simulink model "IM_model"  (R2021a)
settings: Solver=FixedStepAuto  StartTime=0.0  StopTime=40  FixedStep=1e-5  RelTol=1e-3
InitFcn:
  | parameter
values from neighbouring files (symbols this model uses):
  f = 60    [parameter.m]
  Jm = 242.28    [parameter.m]
  L1 = X1/2/pi/f    (= 3.36819606065e-05)    [parameter.m]
  L1a = X1a/2/pi/f    (= 6.73639212131e-05)    [parameter.m]
  L2 = X2/2/pi/f    (= 2.99288217902e-05)    [parameter.m]
  L2a = X2a/2/pi/f    (= 6.41561024441e-05)    [parameter.m]
  Power = 4300e3    (= 4300000)    [parameter.m]
  pp = pole/2    (= 3)    [parameter.m]
  R1 = 0.000789831    [parameter.m]
  R1a = 2*R1    (= 0.001579662)    [parameter.m]
  R2 = 0.00052717    [parameter.m]
  R2a = 2*R2/0.933    (= 0.00113005359057)    [parameter.m]
  Vll = 700    [parameter.m]
libraries: spsACVoltageSourceLib x9, spsFourierLib x3, spsAsynchronousMachineSIUnitsLib x3, spsVoltageMeasurementLib x3, eeStairGenerator x1, spspowerguiLib x1
settings Model: Creator=enes_  LastModifiedBy=enes_

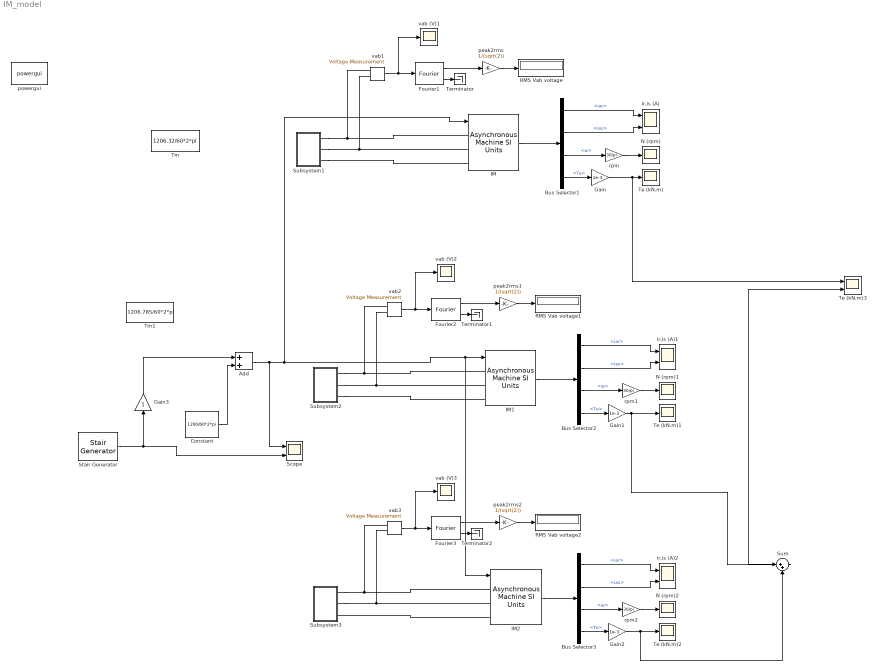
== system IM_model ==
  Add : Sum
  Bus Selector1 : BusSelector  OutputSignals=iar,ias,w,Te
  Bus Selector2 : BusSelector  OutputSignals=iar,ias,w,Te
  Bus Selector3 : BusSelector  OutputSignals=iar,ias,w,Te
  Constant : Constant  Value=1200/60*2*pi
  Fourier1 : spsFourierLib/Fourier  Freq=60  n=1  InInit=[0, 0]  Ts=0
      settings: SourceProductBaseCode=PS
  Fourier2 : spsFourierLib/Fourier  Freq=60  n=1  InInit=[0, 0]  Ts=0
      settings: SourceProductBaseCode=PS
  Fourier3 : spsFourierLib/Fourier  Freq=60  n=1  InInit=[0, 0]  Ts=0
      settings: SourceProductBaseCode=PS
  Gain : Gain  Gain=1e-3
  Gain1 : Gain  Gain=1e-3
  Gain2 : Gain  Gain=1e-3
  Gain3 : Gain
  IM : spsAsynchronousMachineSIUnitsLib/Asynchronous Machine SI Units  RotorType=Squirrel-cage  PresetModel=No  MechanicalLoad=Speed w  ShowDetailedParameters=on  ReferenceFrame=Stationary  Units=SI  MeasurementBus=on  NominalParameters=[Power Vll f]  VoltageRatio=1  Stator=[R1 L1]  Rotor=[R2 L2]  Cage1=[ 0.022 0.226/377]  Cage2=[ 0.022 0.226/377]  Lm=Lm  Mechanical=[Jm 0 pp]  PolePairs=pp  InitialConditions="[ 1,0   0,0,0   0,0,0 ]"  SimulateSaturation=off  Saturation=[14.03593122, 27.81365428, 53.79336849, 72.68890987, 97.98006896, 148.6815601, 215.7428561, 302.9841135, 428.7778367 ; 230, 322, 414, 460, 506, 552, 598, 644, 690]  LoadFlowParameters=0  TsPowergui=0  TsBlock=-1  IterativeModel=Trapezoidal non iterative  IterativeDiscreteModel=Trapezoidal non iterative  Pmec=0
      settings: AttributesFormatString=\n
  IM1 : spsAsynchronousMachineSIUnitsLib/Asynchronous Machine SI Units  RotorType=Squirrel-cage  PresetModel=No  MechanicalLoad=Speed w  ShowDetailedParameters=on  ReferenceFrame=Stationary  Units=SI  MeasurementBus=on  NominalParameters=[Power/2 Vll f]  VoltageRatio=1  Stator=[R1a L1a]  Rotor=[R2a L2a]  Cage1=[ 0.022 0.226/377]  Cage2=[ 0.022 0.226/377]  Lm=Lma  Mechanical=[Jm 0 pp]  PolePairs=pp  InitialConditions="[ 1,0   0,0,0   0,0,0 ]"  SimulateSaturation=off  Saturation=[14.03593122, 27.81365428, 53.79336849, 72.68890987, 97.98006896, 148.6815601, 215.7428561, 302.9841135, 428.7778367 ; 230, 322, 414, 460, 506, 552, 598, 644, 690]  LoadFlowParameters=0  TsPowergui=0  TsBlock=-1  IterativeModel=Trapezoidal non iterative  IterativeDiscreteModel=Trapezoidal non iterative  Pmec=0
      settings: AttributesFormatString=\n
  IM2 : spsAsynchronousMachineSIUnitsLib/Asynchronous Machine SI Units  RotorType=Squirrel-cage  PresetModel=No  MechanicalLoad=Speed w  ShowDetailedParameters=on  ReferenceFrame=Stationary  Units=SI  MeasurementBus=on  NominalParameters=[Power/2 Vll f]  VoltageRatio=1  Stator=[R1a L1a]  Rotor=[R2a L2a]  Cage1=[ 0.022 0.226/377]  Cage2=[ 0.022 0.226/377]  Lm=Lma  Mechanical=[Jm 0 pp]  PolePairs=pp  InitialConditions="[ 1,0   0,0,0   0,0,0 ]"  SimulateSaturation=off  Saturation=[14.03593122, 27.81365428, 53.79336849, 72.68890987, 97.98006896, 148.6815601, 215.7428561, 302.9841135, 428.7778367 ; 230, 322, 414, 460, 506, 552, 598, 644, 690]  LoadFlowParameters=0  TsPowergui=0  TsBlock=-1  IterativeModel=Trapezoidal non iterative  IterativeDiscreteModel=Trapezoidal non iterative  Pmec=0
      settings: AttributesFormatString=\n
  N (rpm) : Scope
  N (rpm)1 : Scope
  N (rpm)2 : Scope
  RMS Vab voltage : Display
      settings: Decimation=100
  RMS Vab voltage1 : Display
      settings: Decimation=100
  RMS Vab voltage2 : Display
      settings: Decimation=100
  Scope : Scope  NumInputPorts=2
  Stair Generator : eeStairGenerator/Stair Generator  LabelModeActiveChoice=Discrete  TimeInput=1:1:40  AmplitudeInput=1:1:40  SampleTime=1e-5  RepeatPattern=off  OutDataTypeStr=double
      settings: SourceProductBaseCode=PS
  Subsystem1 : Subsystem
  Subsystem2 : Subsystem
  Subsystem3 : Subsystem
  Sum : Sum  Inputs=|++
  Te (kN.m) : Scope
  Te (kN.m)1 : Scope
  Te (kN.m)2 : Scope
  Te (kN.m)3 : Scope  NumInputPorts=2
  Terminator : Terminator
  Terminator1 : Terminator
  Terminator2 : Terminator
  Tm : Constant  Value=1206.32/60*2*pi
  Tm1 : Constant  Value=1206.785/60*2*pi
  ir,is (A) : Scope  NumInputPorts=2
  ir,is (A)1 : Scope  NumInputPorts=2
  ir,is (A)2 : Scope  NumInputPorts=2
  peak2rms : Gain  Gain=1/(sqrt(2))  SaturateOnIntegerOverflow=on  OutDataTypeStr=Inherit: Same as input  ParamDataTypeStr=Inherit: Same as input
  peak2rms1 : Gain  Gain=1/(sqrt(2))  SaturateOnIntegerOverflow=on  OutDataTypeStr=Inherit: Same as input  ParamDataTypeStr=Inherit: Same as input
  peak2rms2 : Gain  Gain=1/(sqrt(2))  SaturateOnIntegerOverflow=on  OutDataTypeStr=Inherit: Same as input  ParamDataTypeStr=Inherit: Same as input
  powergui : spspowerguiLib/powergui  SimulationMode=Continuous  SampleTime=0  frequency=60  Iterations=50  frequencyindice=60  Pbase=100e6  ErrMax=1e-4  UnitsV=kV  UnitsW=MW  buscounter=0  FunctionMessages=off  echomessages=off  EnableUseOfTLC=off  CurrentSourceSwitches=off  DisableSnubberDevices=off  DisableRonSwitches=off  DisableVfSwitches=off  DisplayEquations=off  AutomaticDiscreteSolvers=off  SolverType=Tustin  Interpol=off  ExternalGateDelay=off  methode=off  Ts=0  x0status=blocks  SPID=on  SwTol=0  HookPort=off  NonlinearTolerance=1e-4  nMaxIteration=100  ContinueOnMaxIteration=off  RestoreLinks=warning  ResistiveCurrentMeasurement=off  Frange=[0:2:500]  Ylog=off  Xlog=on  ShowGrid=off  save=off  variable=ZData  structure=0  ZoomFFT=on  StartTime=0.0  cycles=1  DisplayStyle=1  fundamental=60  FreqAxis=off  MaxFrequency=1000  frequencyindicesteady=1  RmsSteady=1  display=off
  rpm : Gain  Gain=30/pi  SaturateOnIntegerOverflow=on  OutDataTypeStr=Inherit: Same as input  ParamDataTypeStr=Inherit: Same as input
  rpm1 : Gain  Gain=30/pi  SaturateOnIntegerOverflow=on  OutDataTypeStr=Inherit: Same as input  ParamDataTypeStr=Inherit: Same as input
  rpm2 : Gain  Gain=30/pi  SaturateOnIntegerOverflow=on  OutDataTypeStr=Inherit: Same as input  ParamDataTypeStr=Inherit: Same as input
  vab (V)1 : Scope
  vab (V)2 : Scope
  vab (V)3 : Scope
  vab1 : spsVoltageMeasurementLib/Voltage Measurement  Tag=PoWeRsYsTeMmEaSuReMeNt  PhasorSimulation=off  OutputType=Magnitude  PSBequivalent=0
  vab2 : spsVoltageMeasurementLib/Voltage Measurement  Tag=PoWeRsYsTeMmEaSuReMeNt  PhasorSimulation=off  OutputType=Magnitude  PSBequivalent=0
  vab3 : spsVoltageMeasurementLib/Voltage Measurement  Tag=PoWeRsYsTeMmEaSuReMeNt  PhasorSimulation=off  OutputType=Magnitude  PSBequivalent=0
  wires:
  Bus Selector1/3 -> rpm/1  "<w>"
  Bus Selector1/1 -> ir,is (A)/1  "<iar>"
  IM/1 -> Bus Selector1/1
  Bus Selector1/4 -> Gain/1  "<Te>"
  Fourier1/2 -> Terminator/1
  vab1/1 -> Fourier1/1, vab (V)1/1
  rpm/1 -> N (rpm)/1
  Fourier1/1 -> peak2rms/1
  peak2rms/1 -> RMS Vab voltage/1
  Bus Selector1/2 -> ir,is (A)/2  "<ias>"
  Gain/1 -> Te (kN.m)3/1, Te (kN.m)/1
  Gain1/1 -> Sum/1, Te (kN.m)1/1
  Bus Selector2/2 -> ir,is (A)1/2  "<ias>"
  rpm1/1 -> N (rpm)1/1
  Fourier2/1 -> peak2rms1/1
  vab2/1 -> Fourier2/1, vab (V)2/1
  Fourier2/2 -> Terminator1/1
  Bus Selector2/1 -> ir,is (A)1/1  "<iar>"
  Bus Selector2/4 -> Gain1/1  "<Te>"
  IM1/1 -> Bus Selector2/1
  peak2rms1/1 -> RMS Vab voltage1/1
  Bus Selector2/3 -> rpm1/1  "<w>"
  Bus Selector3/3 -> rpm2/1  "<w>"
  IM2/1 -> Bus Selector3/1
  Bus Selector3/1 -> ir,is (A)2/1  "<iar>"
  Fourier3/2 -> Terminator2/1
  peak2rms2/1 -> RMS Vab voltage2/1
  Fourier3/1 -> peak2rms2/1
  Bus Selector3/4 -> Gain2/1  "<Te>"
  Bus Selector3/2 -> ir,is (A)2/2  "<ias>"
  Gain2/1 -> Sum/2, Te (kN.m)2/1
  rpm2/1 -> N (rpm)2/1
  Add/1 -> Scope/1, IM2/1, IM1/1, IM/1
  vab3/1 -> Fourier3/1, vab (V)3/1
  Sum/1 -> Te (kN.m)3/2
  Stair Generator/1 -> Scope/2, Gain3/1
  Gain3/1 -> Add/1
  Constant/1 -> Add/2
  connections:
  Subsystem1/RConn1 -- vab1/LConn1 -- IM/LConn1
  Subsystem1/RConn2 -- vab1/LConn2 -- IM/LConn2
  Subsystem1/RConn3 -- IM/LConn3
  Subsystem2/RConn2 -- vab2/LConn2 -- IM1/LConn2
  Subsystem2/RConn1 -- vab2/LConn1 -- IM1/LConn1
  Subsystem2/RConn3 -- IM1/LConn3
  Subsystem3/RConn1 -- IM2/LConn1 -- vab3/LConn1
  Subsystem3/RConn2 -- IM2/LConn2 -- vab3/LConn2
  IM2/LConn3 -- Subsystem3/RConn3

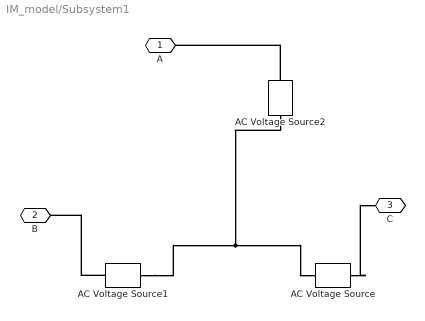
== system IM_model/Subsystem1 ==
  AC Voltage Source : spsACVoltageSourceLib/AC Voltage Source  Amplitude=Vll/sqrt(3)*sqrt(2)  Phase=120  Frequency=f  SampleTime=0  Measurements=None  BusType=swing  Pref=10e3  Qref=0  Qmin=-inf  Qmax=+inf
  AC Voltage Source1 : spsACVoltageSourceLib/AC Voltage Source  Amplitude=Vll/sqrt(3)*sqrt(2)  Phase=240  Frequency=f  SampleTime=0  Measurements=None  BusType=swing  Pref=10e3  Qref=0  Qmin=-inf  Qmax=+inf
  AC Voltage Source2 : spsACVoltageSourceLib/AC Voltage Source  Amplitude=Vll/sqrt(3)*sqrt(2)  Phase=0  Frequency=f  SampleTime=0  Measurements=None  BusType=swing  Pref=10e3  Qref=0  Qmin=-inf  Qmax=+inf
  A : PMIOPort  Side=Right
  B : PMIOPort  Port=2  Side=Right
  C : PMIOPort  Port=3  Side=Right
  connections:
  AC Voltage Source2/LConn1 -- AC Voltage Source1/LConn1 -- AC Voltage Source/LConn1
  AC Voltage Source1/RConn1 -- B/RConn1
  AC Voltage Source2/RConn1 -- A/RConn1
  AC Voltage Source/RConn1 -- C/RConn1

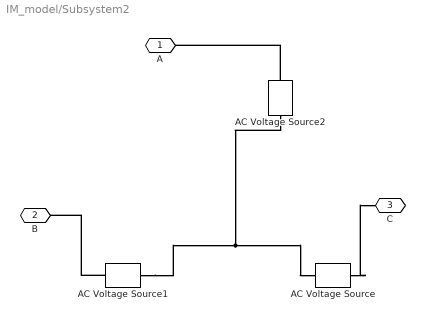
== system IM_model/Subsystem2 ==
  AC Voltage Source : spsACVoltageSourceLib/AC Voltage Source  Amplitude=Vll/sqrt(3)*sqrt(2)  Phase=120  Frequency=f  SampleTime=0  Measurements=None  BusType=swing  Pref=10e3  Qref=0  Qmin=-inf  Qmax=+inf
  AC Voltage Source1 : spsACVoltageSourceLib/AC Voltage Source  Amplitude=Vll/sqrt(3)*sqrt(2)  Phase=240  Frequency=f  SampleTime=0  Measurements=None  BusType=swing  Pref=10e3  Qref=0  Qmin=-inf  Qmax=+inf
  AC Voltage Source2 : spsACVoltageSourceLib/AC Voltage Source  Amplitude=Vll/sqrt(3)*sqrt(2)  Phase=0  Frequency=f  SampleTime=0  Measurements=None  BusType=swing  Pref=10e3  Qref=0  Qmin=-inf  Qmax=+inf
  A : PMIOPort  Side=Right
  B : PMIOPort  Port=2  Side=Right
  C : PMIOPort  Port=3  Side=Right
  connections:
  AC Voltage Source2/LConn1 -- AC Voltage Source1/LConn1 -- AC Voltage Source/LConn1
  AC Voltage Source1/RConn1 -- B/RConn1
  AC Voltage Source2/RConn1 -- A/RConn1
  AC Voltage Source/RConn1 -- C/RConn1

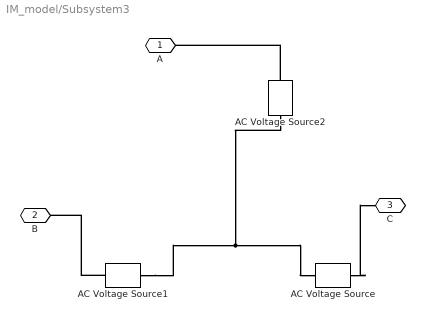
== system IM_model/Subsystem3 ==
  AC Voltage Source : spsACVoltageSourceLib/AC Voltage Source  Amplitude=Vll/sqrt(3)*sqrt(2)  Phase=120  Frequency=f  SampleTime=0  Measurements=None  BusType=swing  Pref=10e3  Qref=0  Qmin=-inf  Qmax=+inf
  AC Voltage Source1 : spsACVoltageSourceLib/AC Voltage Source  Amplitude=Vll/sqrt(3)*sqrt(2)  Phase=240  Frequency=f  SampleTime=0  Measurements=None  BusType=swing  Pref=10e3  Qref=0  Qmin=-inf  Qmax=+inf
  AC Voltage Source2 : spsACVoltageSourceLib/AC Voltage Source  Amplitude=Vll/sqrt(3)*sqrt(2)  Phase=0  Frequency=f  SampleTime=0  Measurements=None  BusType=swing  Pref=10e3  Qref=0  Qmin=-inf  Qmax=+inf
  A : PMIOPort  Side=Right
  B : PMIOPort  Port=2  Side=Right
  C : PMIOPort  Port=3  Side=Right
  connections:
  AC Voltage Source2/LConn1 -- AC Voltage Source1/LConn1 -- AC Voltage Source/LConn1
  AC Voltage Source1/RConn1 -- B/RConn1
  AC Voltage Source2/RConn1 -- A/RConn1
  AC Voltage Source/RConn1 -- C/RConn1
